simulink model "MCU_vectorControl_dsPIC33CK_LVMC"  (R2023a)
settings: Solver=FixedStepDiscrete  StartTime=0.0  StopTime=10.0  FixedStep=5e-5  RelTol=1e-3  EnableMultiTasking=on
undefined symbols (not defined in the file or in its folder): A0, A4, AN0, AN1, B0, B2, Bias1, Bias2, C12, C13, C14, C7, control, D11, D12, D13, D14, D5, D6, D7, diff, DiscIntNeverNeededParam, inverter, Max, MaxPer, model, ms, NumBits1, NumBits2, P20, P32, P55, P60, P61, P62, P69, P70, P71, P75, P76, P77, P78, Pin, pmsm, PosRange1, PosRange2, PWM1max, Resol, s, Slope1, Slope2, us
libraries: simulink x47, MCHP_Blockset x24
(part 3 of 4)

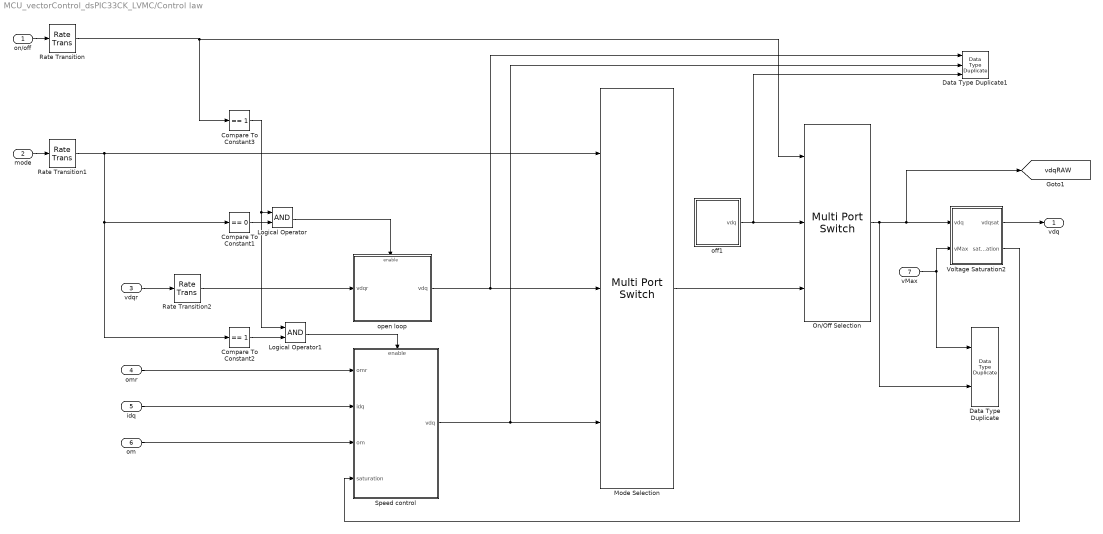
== system MCU_vectorControl_dsPIC33CK_LVMC/Control law ==
  on/off : Inport
  mode : Inport  Port=2
  vdqr : Inport  Port=3
  omr : Inport  Port=4
  idq : Inport  Port=5
  om : Inport  Port=6
  vMax : Inport  Port=7
  Compare To Constant1 : simulink/Logic and Bit Operations/Compare To Constant  relop===  const=0  OutDataTypeStr=boolean
  Compare To Constant2 : simulink/Logic and Bit Operations/Compare To Constant  relop===  const=1  OutDataTypeStr=boolean
  Compare To Constant3 : simulink/Logic and Bit Operations/Compare To Constant  relop===  const=1  OutDataTypeStr=boolean
  Data Type Duplicate : DataTypeDuplicate
  Data Type Duplicate1 : DataTypeDuplicate  NumInputPorts=3
  Logical Operator : Logic  AllPortsSameDT=off  OutDataTypeStr=boolean
  Logical Operator1 : Logic  AllPortsSameDT=off  OutDataTypeStr=boolean
  Mode Selection : MultiPortSwitch  DataPortOrder=Zero-based contiguous  Inputs=2  DiagnosticForDefault=None  zeroidx=on  SaturateOnIntegerOverflow=off  InputSameDT=off
  On/Off Selection : MultiPortSwitch  DataPortOrder=Zero-based contiguous  Inputs=2  DiagnosticForDefault=None  zeroidx=on  SaturateOnIntegerOverflow=off  InputSameDT=off
  Rate Transition : RateTransition
  Rate Transition1 : RateTransition
  Rate Transition2 : RateTransition
  Speed control : Subsystem
      settings: LibrarySourceBlock=insa_control_base/Current Control  PortSchema="{\"entries\":[{\"content\":{\"sides\":[{\"content\":{\"connectorIds\":[\"In1\",\"In2\",\"In3\",\"In4\"]},\"type\":\"ConnectorPlacement.EquallySpacedRectSide\",\"uuid\":\"e7aaa2d5-acdd-4a4d-91b1-423dc6f26e4f\"},{\"content\":{\"connectorIds\":[\"Out1\"],\"side\":\"RIGHT\"},\"type\":\"ConnectorPlacement.EquallySpacedRectSide\",\"uuid\":\"81691e4d-c138-404c-a913-2433211e99ad\"},{\"content\":{\"connectorIds\":[\"In5\"],\"side\":\"TOP\"},\"type\":\"ConnectorPlacement.EquallySpacedRectSide\",\"uuid\":\"67eaf657-96ad-4741-9677-f3dc17f9f096\"}]},\"type\":\"ConnectorPlacement.EquallySpacedConnector\",\"uuid\":\"09d68ba6-6bd5-4801-b033-56cd43b3cecf\"}],\"packageUris\":[\"http://schema.mathworks.com/mf0/Connector/R2020b\"],\"version\":\"1.0\"}"
  Voltage Saturation2 : Subsystem
  off1 : Subsystem
  open loop : Subsystem
  vdq : Outport  VectorParamsAs1DForOutWhenUnconnected=off
  tag scope: vdqRAW=global
  wires:
  Speed control/1(vdq) -> Data Type Duplicate1/2, Mode Selection/3
  Voltage Saturation2/2(saturation) -> Speed control/4(saturation)
  idq/1 -> Speed control/2(idq)
  om/1 -> Speed control/3(om)
  Logical Operator1/1 -> Speed control/5(enable)
  Compare To Constant3/1 -> Logical Operator/1, Logical Operator1/1
  Compare To Constant1/1 -> Logical Operator/2
  vdqr/1 -> Rate Transition2/1
  on/off/1 -> Rate Transition/1
  open loop/1(vdq) -> Mode Selection/2, Data Type Duplicate1/1
  off1/1(vdq) -> Data Type Duplicate1/3, On/Off Selection/2
  Mode Selection/1 -> On/Off Selection/3
  On/Off Selection/1 -> [vdqRAW], Voltage Saturation2/1(vdq), Data Type Duplicate/2
  vMax/1 -> Data Type Duplicate/1, Voltage Saturation2/2(vMax)
  Logical Operator/1 -> open loop/Enable
  Compare To Constant2/1 -> Logical Operator1/2
  mode/1 -> Rate Transition1/1
  Voltage Saturation2/1(vdqsat) -> vdq/1
  Rate Transition/1 -> Compare To Constant3/1, On/Off Selection/1
  Rate Transition1/1 -> Mode Selection/1, Compare To Constant2/1, Compare To Constant1/1
  Rate Transition2/1 -> open loop/1(vdqr)
  omr/1 -> Speed control/1(omr)

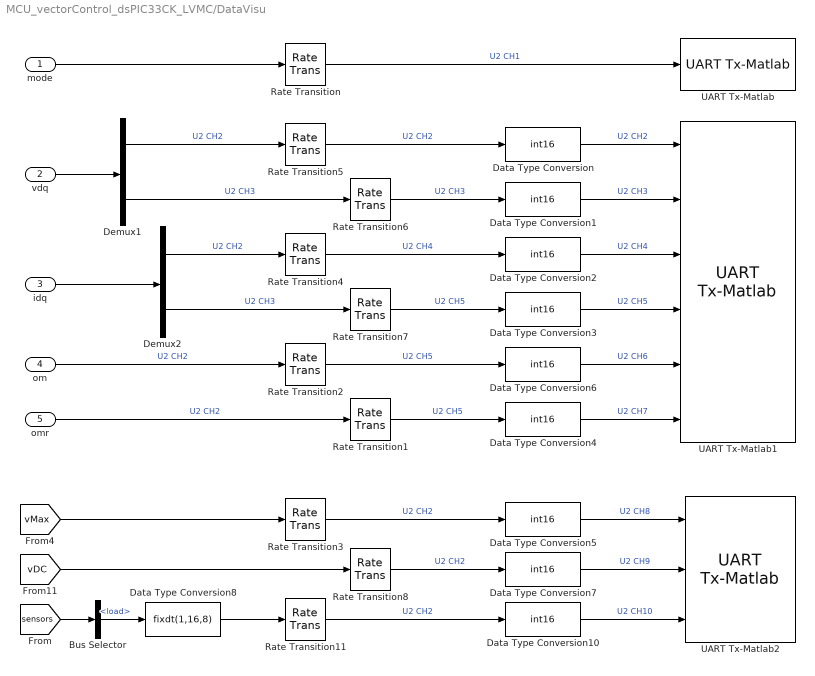
== system MCU_vectorControl_dsPIC33CK_LVMC/DataVisu ==
  mode : Inport
  vdq : Inport  Port=2
  idq : Inport  Port=3
  om : Inport  Port=4
  omr : Inport  Port=5
  Bus Selector : BusSelector  OutputSignals=MCU.load
  Data Type Conversion{,1..7,10} (9 alike) : DataTypeConversion  OutDataTypeStr=int16  ConvertRealWorld=Stored Integer (SI)  SaturateOnIntegerOverflow=off  RndMeth=Floor
  Data Type Conversion8 : DataTypeConversion  OutDataTypeStr=fixdt(1,16,8)  SaturateOnIntegerOverflow=off  RndMeth=Floor
  Demux1 : Demux  Outputs=2
  Demux2 : Demux  Outputs=2
  Rate Transition{,1..8,11} (10 alike) : RateTransition
  UART Tx-Matlab : MCHP_Blockset/BUS UART/UART Tx-Matlab  UART_REF=2  CHANNELS=[1]  AllOrNothing=off  SampleTime=.01  MCHP_MASTERLINK=MCU_vectorControl_dsPIC33CK_LVMC/BOARD dsPIC33CK LVMC/Microchip Master  MCHP_COMPILED_INFO="CompiledSampleTime= [0.010000000000000000208   0 ];CompiledInportDataTypes=[  5 ];CompiledInportDataWidth=[1];"
      settings: SourceProductName=MPLAB Device Blocks for Simulink
  UART Tx-Matlab1 : MCHP_Blockset/BUS UART/UART Tx-Matlab  UART_REF=2  CHANNELS=[2:7]  AllOrNothing=off  SampleTime=0.0005  MCHP_MASTERLINK=MCU_vectorControl_dsPIC33CK_LVMC/BOARD dsPIC33CK LVMC/Microchip Master  MCHP_COMPILED_INFO="CompiledSampleTime= [0.00050000000000000001041   0 ];CompiledInportDataTypes=[  4   4   4   4   4   4 ];CompiledInportDataWidth=[1  1  1  1  1  1];"
      settings: SourceProductName=MPLAB Device Blocks for Simulink
  UART Tx-Matlab2 : MCHP_Blockset/BUS UART/UART Tx-Matlab  UART_REF=2  CHANNELS=[8:10]  AllOrNothing=off  SampleTime=.01  MCHP_MASTERLINK=MCU_vectorControl_dsPIC33CK_LVMC/BOARD dsPIC33CK LVMC/Microchip Master  MCHP_COMPILED_INFO="CompiledSampleTime= [0.010000000000000000208   0 ];CompiledInportDataTypes=[  4   4   4 ];CompiledInportDataWidth=[1  1  1];"
      settings: SourceProductName=MPLAB Device Blocks for Simulink
  wires:
  Data Type Conversion8/1 -> Rate Transition11/1
  [sensors] -> Bus Selector/1
  Rate Transition11/1 -> Data Type Conversion10/1  "U2 CH2"
  Data Type Conversion10/1 -> UART Tx-Matlab2/3  "U2 CH10"
  Bus Selector/1 -> Data Type Conversion8/1  "<load>"
  Rate Transition8/1 -> Data Type Conversion7/1  "U2 CH2"
  Rate Transition3/1 -> Data Type Conversion5/1  "U2 CH2"
  Data Type Conversion7/1 -> UART Tx-Matlab2/2  "U2 CH9"
  Data Type Conversion5/1 -> UART Tx-Matlab2/1  "U2 CH8"
  [vMax] -> Rate Transition3/1
  [vDC] -> Rate Transition8/1
  Rate Transition1/1 -> Data Type Conversion4/1  "U2 CH5"
  Data Type Conversion4/1 -> UART Tx-Matlab1/6  "U2 CH7"
  omr/1 -> Rate Transition1/1  "U2 CH2"
  mode/1 -> Rate Transition/1
  Rate Transition/1 -> UART Tx-Matlab/1  "U2 CH1"
  om/1 -> Rate Transition2/1  "U2 CH2"
  Data Type Conversion6/1 -> UART Tx-Matlab1/5  "U2 CH6"
  Rate Transition2/1 -> Data Type Conversion6/1  "U2 CH5"
  Data Type Conversion3/1 -> UART Tx-Matlab1/4  "U2 CH5"
  Data Type Conversion2/1 -> UART Tx-Matlab1/3  "U2 CH4"
  Data Type Conversion1/1 -> UART Tx-Matlab1/2  "U2 CH3"
  Data Type Conversion/1 -> UART Tx-Matlab1/1  "U2 CH2"
  Rate Transition7/1 -> Data Type Conversion3/1  "U2 CH5"
  Demux1/1 -> Rate Transition5/1  "U2 CH2"
  Rate Transition4/1 -> Data Type Conversion2/1  "U2 CH4"
  Rate Transition6/1 -> Data Type Conversion1/1  "U2 CH3"
  Demux1/2 -> Rate Transition6/1  "U2 CH3"
  Rate Transition5/1 -> Data Type Conversion/1  "U2 CH2"
  Demux2/1 -> Rate Transition4/1  "U2 CH2"
  Demux2/2 -> Rate Transition7/1  "U2 CH3"
  idq/1 -> Demux2/1
  vdq/1 -> Demux1/1

== system MCU_vectorControl_dsPIC33CK_LVMC/Heart-beat 5Hz Blinking ==
  Delay : Delay  DelayLength=1  InitialCondition=0  SampleTime=.1
  Logical Operator : Logic  Operator=NOT  AllPortsSameDT=off  OutDataTypeStr=boolean
  Rate Transition2 : RateTransition  Deterministic=off  OutPortSampleTime=0.01
  LED1 : Outport  VectorParamsAs1DForOutWhenUnconnected=off
  wires:
  Rate Transition2/1 -> LED1/1
  Logical Operator/1 -> Rate Transition2/1, Delay/1
  Delay/1 -> Logical Operator/1

== system MCU_vectorControl_dsPIC33CK_LVMC/Init Enc ==
  rho_cont : Inport
  Constant1 : Constant  Value=[0.5 0.5 0.5]  OutDataTypeStr=Inherit: Inherit via back propagation
  Constant2 : Constant  Value=[.6 .5 .5]  OutDataTypeStr=Inherit: Inherit via back propagation
  Data Type Duplicate : DataTypeDuplicate
  Rate Transition1 : RateTransition
  Rate Transition2 : RateTransition
  Rate Transition3 : RateTransition
  Switch : Switch  Criteria=u2 > Threshold  SaturateOnIntegerOverflow=off  InputSameDT=off
  Switch1 : Switch  Criteria=u2 > Threshold  SaturateOnIntegerOverflow=off  InputSameDT=off
  Wait 1s : Subsystem
  reset encoder : Outport
  PWM [0 1] : Outport  Port=2
  wires:
  Rate Transition2/1 -> Switch/2
  Rate Transition1/1 -> reset encoder/1
  Switch1/1 -> PWM [0 1]/1
  Constant1/1 -> Switch1/3
  Constant2/1 -> Switch/3
  Wait 1s/2(init done) -> Rate Transition2/1
  Switch/1 -> Data Type Duplicate/2, Switch1/1
  rho_cont/1 -> Switch/1, Data Type Duplicate/1
  Wait 1s/1(init enc) -> Rate Transition1/1
  [onoff] -> Wait 1s/Enable, Rate Transition3/1
  Rate Transition3/1 -> Switch1/2

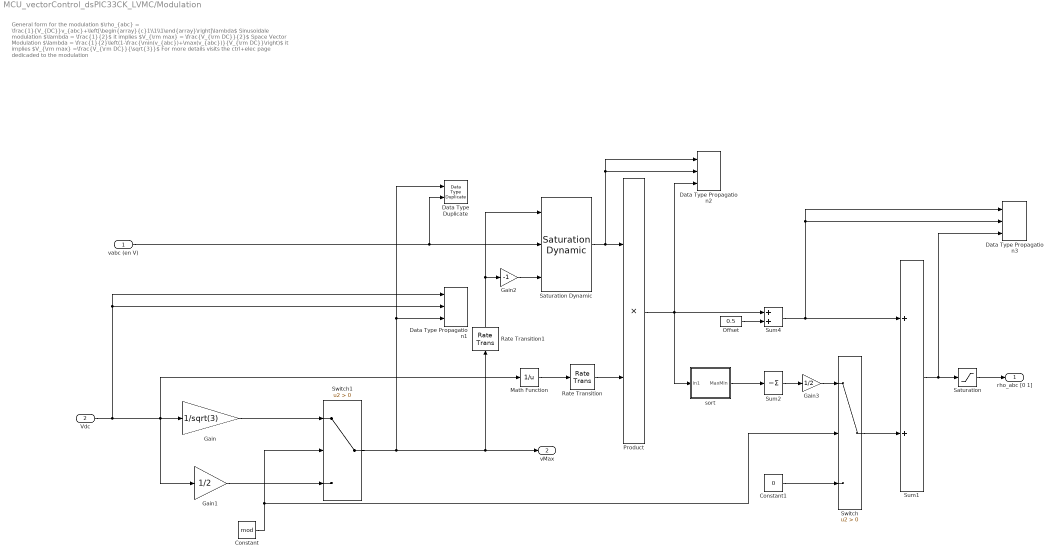
== system MCU_vectorControl_dsPIC33CK_LVMC/Modulation ==
  note: General form for the modulation
      | $\rho_{abc} = \frac{1}{V_{DC}}v_{abc}+\left[\begin{array}{c}1\\1\\1\end{array}\right]\lambda$
      | Sinusoidale modulation
      | $\lambda = \frac{1}{2}$ it implies $V_{\rm max} = \frac{V_{\rm DC}}{2}$
      | Space Vector Modulation
      | $\lambda = \frac{1}{2}\left(1-\frac{\min(v_{abc})+\max(v_{abc})}{V_{\rm DC}}\right)$ it implies $V_{\rm max} =\frac{V_{\rm DC}}{\sqrt{3}}$
      | For more details visits the ctrl+elec page dedicaded to the modulation
  "vabc (en V) " : Inport
  Vdc : Inport  Port=2
  Constant : Constant  Value=mod  OutDataTypeStr=boolean
  Constant1 : Constant  Value=0  OutDataTypeStr=Inherit: Inherit via back propagation
  Data Type Duplicate : DataTypeDuplicate
  Data Type Propagation1 : simulink/Signal Attributes/Data Type Propagation  PropDataType=fixdt(1, 16)  IfRefDouble=double  IfRefSingle=single  IsSigned=TRUE  NumBitsBase=max([NumBits1 NumBits2])  NumBitsMult=1  NumBitsAdd=0  NumBitsAllowFinal=[1:128]  PropScaling=2^-(15-ceil(log2(inverter.vDC/sqrt(3))))  ValuesUsedBestPrec=[100 -100]  SlopeBase=max([PosRange1 PosRange2])  SlopeMult=1/sqrt(3)  SlopeAdd=0  BiasBase=Bias1  BiasMult=1  BiasAdd=0
  Data Type Propagation2 : simulink/Signal Attributes/Data Type Propagation  PropDataType=fixdt(1, 16)  IfRefDouble=double  IfRefSingle=single  IsSigned=TRUE  NumBitsBase=max([NumBits1 NumBits2])  NumBitsMult=1  NumBitsAdd=0  NumBitsAllowFinal=[1:128]  PropScalingMode=Specify via dialog  PropScaling=2^-14  ValuesUsedBestPrec=[100 -100]  SlopeBase=Slope1/Slope2  SlopeMult=1  SlopeAdd=0  BiasBase=Bias1  BiasMult=1  BiasAdd=0
  Data Type Propagation3 : simulink/Signal Attributes/Data Type Propagation  PropDataType=fixdt(1, 16)  IfRefDouble=double  IfRefSingle=single  IsSigned=FALSE  NumBitsBase=max([NumBits1 NumBits2])  NumBitsMult=1  NumBitsAdd=0  NumBitsAllowFinal=[1:128]  PropScalingMode=Specify via dialog  PropScaling=2^-14  ValuesUsedBestPrec=[100 -100]  SlopeBase=Slope1/Slope2  SlopeMult=1  SlopeAdd=0  BiasBase=Bias1  BiasMult=1  BiasAdd=0
  Gain : Gain  Gain=1/sqrt(3)  OutDataTypeStr=Inherit: Same as input
  Gain1 : Gain  Gain=1/2  OutDataTypeStr=Inherit: Same as input
  Gain2 : Gain  Gain=-1  ParamDataTypeStr=int16  OutDataTypeStr=Inherit: Inherit via back propagation
  Gain3 : Gain  Gain=1/2  OutDataTypeStr=Inherit: Same as input
  Math Function : Math  Operator=reciprocal  OutputSignalType=real  OutDataTypeStr=fixdt(0,16,16)  SaturateOnIntegerOverflow=off
  "Offset " : Constant  Value=0.5  OutMin=[0]  OutMax=[1]  OutDataTypeStr=Inherit: Inherit via back propagation
  Product : Product  Inputs=**  OutDataTypeStr=Inherit: Inherit via back propagation  SaturateOnIntegerOverflow=on
  Rate Transition : RateTransition
  Rate Transition1 : RateTransition
  Saturation : Saturate  UpperLimit=1  LowerLimit=0
  Saturation Dynamic : simulink/Discontinuities/Saturation Dynamic  OutMin=[]  OutMax=[]  OutDataTypeStr=Inherit: Same as second input  OutDataType=fixdt(1, 16)  OutScaling=2^-10  DoSatur=off
  Sum1 : Sum  InputSameDT=on  OutMin=[0]  OutMax=[1]  OutDataTypeStr=Inherit: Inherit via back propagation  SaturateOnIntegerOverflow=on
  Sum2 : Sum  Inputs=-  InputSameDT=on  OutMin=[-1]  OutMax=[1]  SaturateOnIntegerOverflow=on  OutDataTypeStr=Inherit: Same as first input
  Sum4 : Sum  InputSameDT=on  OutMin=[-1]  OutMax=[1]  SaturateOnIntegerOverflow=on  OutDataTypeStr=Inherit: Same as first input
  Switch : Switch  Criteria=u2 > Threshold  SaturateOnIntegerOverflow=off  InputSameDT=off
  Switch1 : Switch  Criteria=u2 > Threshold  OutDataTypeStr=Inherit: Inherit via back propagation  SaturateOnIntegerOverflow=off  InputSameDT=off
  sort : Subsystem
  rho_abc [0 1] : Outport  VectorParamsAs1DForOutWhenUnconnected=off
  vMax : Outport  Port=2  VectorParamsAs1DForOutWhenUnconnected=off
  wires:
  Sum1/1 -> Saturation/1, Data Type Propagation3/3
  Vdc/1 -> Data Type Propagation1/2, Data Type Propagation1/1, Gain/1, Math Function/1, Gain1/1
  Gain3/1 -> Switch/1
  Saturation/1 -> rho_abc [0 1]/1
  Saturation Dynamic/1 -> Product/1, Data Type Propagation2/1, Data Type Propagation2/2
  Gain1/1 -> Switch1/3
  Gain/1 -> Switch1/1
  sort/1(MaxMin) -> Sum2/1
  Sum2/1 -> Gain3/1
  Sum4/1 -> Data Type Propagation3/2, Data Type Propagation3/1, Sum1/1
  Constant1/1 -> Switch/3
  Switch/1 -> Sum1/2
  "Offset "/1 -> Sum4/2
  Product/1 -> Data Type Propagation2/3, Sum4/1, sort/1(In1)
  Gain2/1 -> Saturation Dynamic/3
  Math Function/1 -> Rate Transition/1
  Switch1/1 -> Rate Transition1/1, vMax/1, Data Type Propagation1/3, Data Type Duplicate/1
  Constant/1 -> Switch1/2, Switch/2
  "vabc (en V) "/1 -> Data Type Duplicate/2, Saturation Dynamic/2
  Rate Transition/1 -> Product/2
  Rate Transition1/1 -> Saturation Dynamic/1, Gain2/1

== system MCU_vectorControl_dsPIC33CK_LVMC/Motor Choice + Gain Tunning ==

== system MCU_vectorControl_dsPIC33CK_LVMC/Park ==
  xab(c) : Inport
  P(pth) : Inport  Port=2
  Clarke : Subsystem
  Park : Subsystem
  idq : Outport
  wires:
  P(pth)/1 -> Park/2(P(pth))
  Park/1(xdq) -> idq/1  "idq"
  xab(c)/1 -> Clarke/1(xab(c))
  Clarke/1(xalphabeta) -> Park/1(xalphabeta)

== system MCU_vectorControl_dsPIC33CK_LVMC/Park inverse ==
  xdq : Inport
  P(pth) : Inport  Port=2
  Clarke Inverse : Subsystem
  Park inverse : Subsystem
  xabc : Outport
  wires:
  P(pth)/1 -> Park inverse/2(P(pth))
  Clarke Inverse/1(xabc) -> xabc/1
  xdq/1 -> Park inverse/1(xdq)
  Park inverse/1(xalpahbeta) -> Clarke Inverse/1(xalphabeta)

== system MCU_vectorControl_dsPIC33CK_LVMC/Rot ==
  sin cos : Inport
  Demux3 : Demux  Outputs=2
  Gain : Gain  Gain=-1  OutDataTypeStr=Inherit: Same as input
  Mux1 : Mux
  Reshape : Reshape  OutputDimensionality=Customize  OutputDimensions=[2,2]
  "cos sin -sin cos " : Outport  PortDimensions=[2 2]
  wires:
  Demux3/2 -> Mux1/1, Mux1/4
  Demux3/1 -> Gain/1, Mux1/3
  Mux1/1 -> Reshape/1
  Gain/1 -> Mux1/2
  sin cos/1 -> Demux3/1
  Reshape/1 -> "cos sin -sin cos "/1

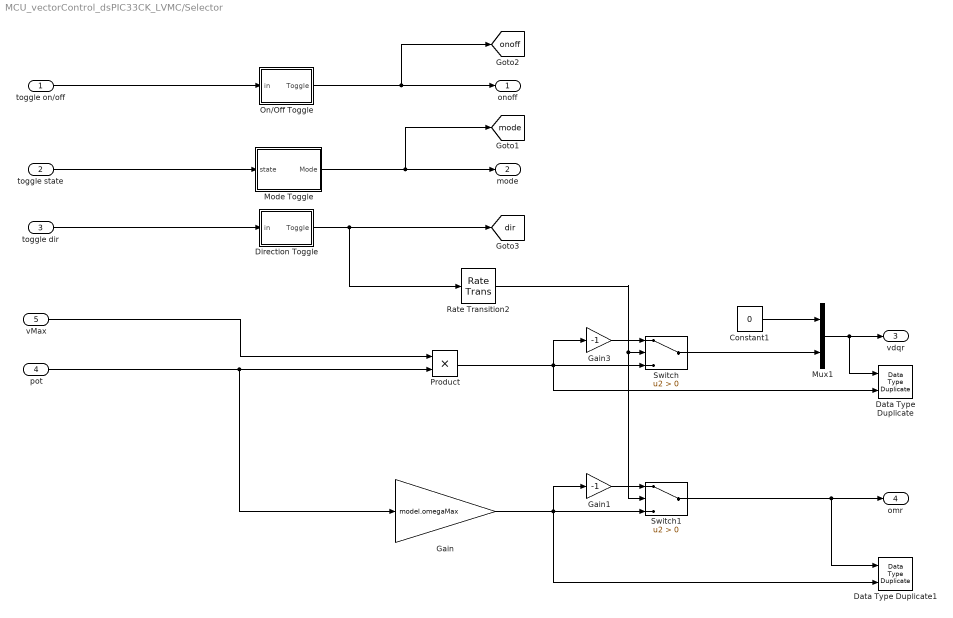
== system MCU_vectorControl_dsPIC33CK_LVMC/Selector ==
  toggle on/off : Inport  SampleTime=.01
  toggle state : Inport  Port=2  SampleTime=.01
  toggle dir : Inport  Port=3  SampleTime=.01
  pot : Inport  Port=4
  vMax : Inport  Port=5
  Constant1 : Constant  Value=0  OutDataTypeStr=Inherit: Inherit via back propagation
  Data Type Duplicate : DataTypeDuplicate
  Data Type Duplicate1 : DataTypeDuplicate
  Direction Toggle : Subsystem
  Gain : Gain  Gain=model.omegaMax  OutDataTypeStr=Inherit: Inherit via back propagation
  Gain1 : Gain  Gain=-1  OutDataTypeStr=Inherit: Inherit via back propagation  SaturateOnIntegerOverflow=on
  Gain3 : Gain  Gain=-1  OutDataTypeStr=Inherit: Inherit via back propagation  SaturateOnIntegerOverflow=on
  Mode Toggle : Subsystem
  Mux1 : Mux  Inputs=2
  On/Off Toggle : Subsystem
  Product : Product  OutDataTypeStr=Inherit: Same as first input
  Rate Transition2 : RateTransition  Integrity=off  OutPortSampleTime=0.001
  Switch : Switch  Criteria=u2 > Threshold  OutDataTypeStr=Inherit: Inherit via back propagation  SaturateOnIntegerOverflow=off  InputSameDT=off
  Switch1 : Switch  Criteria=u2 > Threshold  OutDataTypeStr=Inherit: Inherit via back propagation  SaturateOnIntegerOverflow=off  InputSameDT=off
  onoff : Outport
  mode : Outport  Port=2
  vdqr : Outport  Port=3  VectorParamsAs1DForOutWhenUnconnected=off
  omr : Outport  Port=4  VectorParamsAs1DForOutWhenUnconnected=off
  tag scope: dir=global, mode=global, onoff=global
  wires:
  Switch1/1 -> omr/1, Data Type Duplicate1/1
  Direction Toggle/1(Toggle) -> Rate Transition2/1, [dir]
  Gain1/1 -> Switch1/1
  Gain/1 -> Gain1/1, Switch1/3, Data Type Duplicate1/2
  Product/1 -> Data Type Duplicate/2, Switch/3, Gain3/1
  Mux1/1 -> Data Type Duplicate/1, vdqr/1
  Constant1/1 -> Mux1/1
  toggle on/off/1 -> On/Off Toggle/1(in)
  On/Off Toggle/1(Toggle) -> [onoff], onoff/1
  Mode Toggle/1(Mode) -> [mode], mode/1
  toggle state/1 -> Mode Toggle/1(state)
  toggle dir/1 -> Direction Toggle/1(in)
  Gain3/1 -> Switch/1
  Switch/1 -> Mux1/2
  vMax/1 -> Product/1
  Rate Transition2/1 -> Switch/2, Switch1/2
  pot/1 -> Gain/1, Product/2

== system MCU_vectorControl_dsPIC33CK_LVMC/BOARD dsPIC33CK LVMC/ADC ==
  ADC dsPIC High Speed SAR Motor Currents : MCHP_Blockset/Analog IO/ADC dsPIC High Speed SAR  ACLKCON=Optimized for PWM resolution & ADC conversion speed  ADC_FRACT=Fractional (left aligned)  ADC_NRE=off  DMA_Size=Single trigger - (default)  ADC_Synchronisation=Triggered by custom source  ADC_Trig=Dynamic Options  ADC_Trig_TXT=PWM1 Trigger 1  ADC_TrigTimeStep=Trig model step after all sample from this block are converted  ADC_TrigInfo=0  SampleTime=50e-6  S_INPUT=[]  S_INPUT_Size=[]  S_OUTPUT="[5  5]"  S_OUTPUT_Size="[1  1]"  S_ListCustomDatatype=S.S_ListCustomDatatype={};  MCHP_USER_INTERRUPTS={ADCAN0}{ADCBUF0}{ADC Data 0 Ready}{VectorName(ADCAN0Interrupt) Priority(-1) RegisterReadClear(ADCBUF0)Config_BitSet(ADIELbits.IE0) };{ADCAN1}{ADCBUF1}{ADC Data 1 Ready}{VectorName(ADCAN1Interrupt) Priority(-1) RegisterReadClear(ADCBUF1)Config_BitSet(ADIELbits.IE1) };  MCHP_PORT={Analog Input 0}{AN0}15:2:A0;{Analog Input 1}{AN1}15:2:B2;  MCHP_MASTERLINK=MCU_vectorControl_dsPIC33CK_LVMC/BOARD dsPIC33CK LVMC/Microchip Master  MCHP_CRC=3824902  ADC_Info=Total Time = 640(ns)  ADC0_pin=Dynamic Options  ADC0_pin_TXT=AN0 / A0 / Pin[16]  ADC0_R="< 5    kOhm"  ADC0_res=12 bits  ADC0_signed=signed 16 bits  ADC0_FILTER=No Oversampling  ADC0_FILTER_nSamples=256 samples  ADC0_STRGEN=Start sampling followed by conversion  ADC0_STRGEN_on=Start sampling followed by conversion  ADC0_SSAMPEN=off  ADC0_Info=tSmp_min=260(ns) x 1 = 260(ns) ; tConv=370(ns) x 1 = 370(ns) ; TOTAL=640(ns)  ADC1_pin=Dynamic Options  ADC1_pin_TXT=AN1 / B2 / Pin[41]  ADC1_R="< 5    kOhm"  ADC1_res=12 bits  ADC1_signed=signed 16 bits  ADC1_FILTER=No Oversampling  ADC1_FILTER_nSamples=128 samples  ADC1_STRGEN=Start sampling followed by conversion  ADC1_STRGEN_on=Start sampling followed by conversion  ADC1_SSAMPEN=off  ADC1_Info=tSmp_min=260(ns) x 1 = 260(ns) ; tConv=370(ns) x 1 = 370(ns) ; TOTAL=640(ns)  ADC2_pin=Dynamic Options  ADC2_pin_TXT=Not used  ADC2_R="< 5    kOhm"  ADC2_res=12 bits  ADC2_signed=signed 16 bits  ADC2_FILTER=No Oversampling  ADC2_FILTER_nSamples=256 samples  ADC2_STRGEN=End sampling and start conversion  ADC2_STRGEN_on=Start sampling followed by conversion  ADC2_SSAMPEN=on  ADC2_Info=tSmp_min=14.706(ns) x 0 = 0(s) ; tConv=154.41(ns) x 0 = 0(s) ; TOTAL=0(s)  ADC3_pin=Dynamic Options  ADC3_pin_TXT=Not used  ADC3_R="< 10   kOhm"  ADC3_res=12 bits  ADC3_signed=signed 16 bits  ADC3_FILTER=Burst convert of n samples are Summed  ADC3_FILTER_nSamples=64 samples  ADC3_STRGEN=End sampling and start conversion  ADC3_STRGEN_on=Start sampling followed by conversion  ADC3_SSAMPEN=on  ADC3_Info=tSmp_min=14.706(ns) x 0 = 0(s) ; tConv=154.41(ns) x 0 = 0(s) ; TOTAL=0(s)  ADC4_pin=Dynamic Options  ADC4_pin_TXT=Not used  ADC4_R=< 200 Ohm  ADC4_res=12 bits  ADC4_signed=unsigned 16 bits  ADC4_FILTER=No Oversampling  ADC4_FILTER_nSamples=256 samples  ADC4_STRGEN=End sampling and start conversion  ADC4_STRGEN_on=Start sampling followed by conversion  ADC4_SSAMPEN=off  ADC4_Info=tSmp_min=14.706(ns) x 0 = 0(s) ; tConv=154.41(ns) x 0 = 0(s) ; TOTAL=0(s)  ADC5_pin=Dynamic Options  ADC5_pin_TXT=Not used  ADC5_R=< 200 Ohm  ADC5_res=12 bits  ADC5_signed=unsigned 16 bits  ADC5_FILTER=Burst convert of n samples are Summed  ADC5_FILTER_nSamples=256 samples  ADC5_STRGEN=End sampling and start conversion  ADC5_STRGEN_on=Start sampling followed by conversion  ADC5_SSAMPEN=on  ADC5_Info=tSmp_min=14.706(ns) x 0 = 0(s) ; tConv=154.41(ns) x 0 = 0(s) ; TOTAL=0(s)  ADC6_pin=Dynamic Options  ADC6_pin_TXT=Not used  ADC6_R=< 200 Ohm  ADC6_res=12 bits  ADC6_signed=unsigned 16 bits  ADC6_FILTER=Burst convert of n samples are Summed  ADC6_FILTER_nSamples=256 samples  ADC6_STRGEN=End sampling and start conversion  ADC6_STRGEN_on=Start sampling followed by conversion  ADC6_SSAMPEN=on  ADC6_Info=tSmp_min=14.706(ns) x 0 = 0(s) ; tConv=154.41(ns) x 0 = 0(s) ; TOTAL=0(s)  ADC7_R="< 5    kOhm"  ADC7_res=12 bits  ADC7_AN0=Not used  ADC7_AN1=Not used  ADC7_AN2=Not used  ADC7_AN3=Not used  ADC7_AN4=Not used  ADC7_AN5=Not used  ADC7_AN6=Not used  ADC7_AN7=Not used  ADC7_AN8=Not used  ADC7_AN9=Not used  ADC7_AN10=Not used  ADC7_AN11=Not used  ADC7_AN12=Not used  ADC7_AN13=Not used  ADC7_AN14=Not used  ADC7_AN15=Not used  ADC7_AN16=Not used  ADC7_AN17=Not used  ADC7_AN18=Not used  ADC7_AN19=Not used  ADC7_AN20=Not used  ADC7_AN21=Not used  ADC7_AN22=Not used  ADC7_AN23=Not used  ADC7_AN24=Not used  ADC7_AN25=Not used  ADC7_AN26=Not used  ADC7_AN27=Not used  ADC7_AN28=Not used  ADC7_AN29=Not used  ADC7_AN30=Not used  ADC7_AN31=Not used  IVref=Not used  IVTemp=Not used  ADC7_Info=tSmp_min=20(ns) x 0 = 0(s) ; tConv=210(ns) x 0 = 0(s) ; TOTAL=0(s)
      settings: SourceProductName=MPLAB Device Blocks for Simulink
  ADC dsPIC High Speed SAR others : MCHP_Blockset/Analog IO/ADC dsPIC High Speed SAR  ACLKCON=Not used  ADC_FRACT=Fractional (left aligned)  ADC_NRE=off  DMA_Size=Single trigger - (default)  ADC_Synchronisation=Triggered by custom source  ADC_Trig=Dynamic Options  ADC_Trig_TXT=PWM1 Trigger 1  ADC_TrigTimeStep=None (independant)  ADC_TrigInfo=0  SampleTime=50e-6  S_INPUT=[]  S_INPUT_Size=[]  S_OUTPUT="[5  5]"  S_OUTPUT_Size="[1  1]"  S_ListCustomDatatype=S.S_ListCustomDatatype={};  MCHP_USER_INTERRUPTS={ADCAN3}{ADCBUF3}{ADC Data 3 Ready}{VectorName(ADCAN3Interrupt) Priority(-1) RegisterReadClear(ADCBUF3)Config_BitSet(ADIELbits.IE3) };{ADCAN10}{ADCBUF10}{ADC Data 10 Ready}{VectorName(ADCAN10Interrupt) Priority(-1) RegisterReadClear(ADCBUF10)Config_BitSet(ADIELbits.IE10) };{ADCAN14}{ADCBUF14}{ADC Data 14 Ready}{VectorName(ADCAN14Interrupt) Priority(-1) RegisterReadClear(ADCBUF14)Config_BitSet(ADIELbits.IE14) };  MCHP_PORT={Analog Input 4}{AN4}15:2:A4;{Analog Input 11}{AN11}15:2:B9;{Analog Input 15}{AN15}15:2:C3;  MCHP_MASTERLINK=MCU_vectorControl_dsPIC33CK_LVMC/BOARD dsPIC33CK LVMC/Microchip Master  MCHP_CRC=3970270  ADC_Info=Total Time = 1.98(us)  ADC0_pin=Dynamic Options  ADC0_pin_TXT=Not used  ADC0_R="< 5    kOhm"  ADC0_res=12 bits  ADC0_signed=signed 16 bits  ADC0_FILTER=No Oversampling  ADC0_FILTER_nSamples=256 samples  ADC0_STRGEN=Start sampling followed by conversion  ADC0_STRGEN_on=Start sampling followed by conversion  ADC0_SSAMPEN=off  ADC0_Info=tSmp_min=20(ns) x 0 = 0(s) ; tConv=210(ns) x 0 = 0(s) ; TOTAL=0(s)  ADC1_pin=Dynamic Options  ADC1_pin_TXT=Not used  ADC1_R="< 5    kOhm"  ADC1_res=12 bits  ADC1_signed=signed 16 bits  ADC1_FILTER=No Oversampling  ADC1_FILTER_nSamples=128 samples  ADC1_STRGEN=Start sampling followed by conversion  ADC1_STRGEN_on=Start sampling followed by conversion  ADC1_SSAMPEN=off  ADC1_Info=tSmp_min=20(ns) x 0 = 0(s) ; tConv=210(ns) x 0 = 0(s) ; TOTAL=0(s)  ADC2_pin=Dynamic Options  ADC2_pin_TXT=Not used  ADC2_R="< 5    kOhm"  ADC2_res=12 bits  ADC2_signed=signed 16 bits  ADC2_FILTER=No Oversampling  ADC2_FILTER_nSamples=256 samples  ADC2_STRGEN=End sampling and start conversion  ADC2_STRGEN_on=Start sampling followed by conversion  ADC2_SSAMPEN=on  ADC2_Info=tSmp_min=14.706(ns) x 0 = 0(s) ; tConv=154.41(ns) x 0 = 0(s) ; TOTAL=0(s)  ADC3_pin=Dynamic Options  ADC3_pin_TXT=Not used  ADC3_R="< 10   kOhm"  ADC3_res=12 bits  ADC3_signed=signed 16 bits  ADC3_FILTER=Burst convert of n samples are Summed  ADC3_FILTER_nSamples=64 samples  ADC3_STRGEN=End sampling and start conversion  ADC3_STRGEN_on=Start sampling followed by conversion  ADC3_SSAMPEN=on  ADC3_Info=tSmp_min=14.706(ns) x 0 = 0(s) ; tConv=154.41(ns) x 0 = 0(s) ; TOTAL=0(s)  ADC4_pin=Dynamic Options  ADC4_pin_TXT=Not used  ADC4_R=< 200 Ohm  ADC4_res=12 bits  ADC4_signed=unsigned 16 bits  ADC4_FILTER=No Oversampling  ADC4_FILTER_nSamples=256 samples  ADC4_STRGEN=End sampling and start conversion  ADC4_STRGEN_on=Start sampling followed by conversion  ADC4_SSAMPEN=off  ADC4_Info=tSmp_min=14.706(ns) x 0 = 0(s) ; tConv=154.41(ns) x 0 = 0(s) ; TOTAL=0(s)  ADC5_pin=Dynamic Options  ADC5_pin_TXT=Not used  ADC5_R=< 200 Ohm  ADC5_res=12 bits  ADC5_signed=unsigned 16 bits  ADC5_FILTER=Burst convert of n samples are Summed  ADC5_FILTER_nSamples=256 samples  ADC5_STRGEN=End sampling and start conversion  ADC5_STRGEN_on=Start sampling followed by conversion  ADC5_SSAMPEN=on  ADC5_Info=tSmp_min=14.706(ns) x 0 = 0(s) ; tConv=154.41(ns) x 0 = 0(s) ; TOTAL=0(s)  ADC6_pin=Dynamic Options  ADC6_pin_TXT=Not used  ADC6_R=< 200 Ohm  ADC6_res=12 bits  ADC6_signed=unsigned 16 bits  ADC6_FILTER=Burst convert of n samples are Summed  ADC6_FILTER_nSamples=256 samples  ADC6_STRGEN=End sampling and start conversion  ADC6_STRGEN_on=Start sampling followed by conversion  ADC6_SSAMPEN=on  ADC6_Info=tSmp_min=14.706(ns) x 0 = 0(s) ; tConv=154.41(ns) x 0 = 0(s) ; TOTAL=0(s)  ADC7_R="< 5    kOhm"  ADC7_res=12 bits  ADC7_AN0=Not used  ADC7_AN1=Not used  ADC7_AN2=Not used  ADC7_AN3=Not used  ADC7_AN4=signed int16  ADC7_AN5=Not used  ADC7_AN6=Not used  ADC7_AN7=Not used  ADC7_AN8=Not used  ADC7_AN9=Not used  ADC7_AN10=Not used  ADC7_AN11=unsigned int16  ADC7_AN12=Not used  ADC7_AN13=Not used  ADC7_AN14=Not used  ADC7_AN15=unsigned int16  ADC7_AN16=Not used  ADC7_AN17=Not used  ADC7_AN18=Not used  ADC7_AN19=Not used  ADC7_AN20=Not used  ADC7_AN21=Not used  ADC7_AN22=Not used  ADC7_AN23=Not used  ADC7_AN24=Not used  ADC7_AN25=Not used  ADC7_AN26=Not used  ADC7_AN27=Not used  ADC7_AN28=Not used  ADC7_AN29=Not used  ADC7_AN30=Not used  ADC7_AN31=Not used  IVref=Not used  IVTemp=Not used  ADC7_Info=tSmp_min=280(ns) x 3 = 840(ns) ; tConv=370(ns) x 3 = 1.11(us) ; TOTAL=1.98(us)
      settings: SourceProductName=MPLAB Device Blocks for Simulink
  Ia : Outport  VectorParamsAs1DForOutWhenUnconnected=off
  Ib : Outport  Port=2  VectorParamsAs1DForOutWhenUnconnected=off
  IBus : Outport  Port=3  VectorParamsAs1DForOutWhenUnconnected=off
  pot : Outport  Port=4  VectorParamsAs1DForOutWhenUnconnected=off
  V_BUS : Outport  Port=5  VectorParamsAs1DForOutWhenUnconnected=off
  wires:
  ADC dsPIC High Speed SAR Motor Currents/2 -> Ib/1
  ADC dsPIC High Speed SAR Motor Currents/1 -> Ia/1
  ADC dsPIC High Speed SAR others/1 -> IBus/1
  ADC dsPIC High Speed SAR others/2 -> pot/1
  ADC dsPIC High Speed SAR others/3 -> V_BUS/1

== system MCU_vectorControl_dsPIC33CK_LVMC/BOARD dsPIC33CK LVMC/Center & sign reversal ==
  I_ab : Inport
  Bias Update : Inport  Port=2
  Average and Sign reverse : Sum  Inputs=+-  OutDataTypeStr=Inherit: Same as accumulator  SaturateOnIntegerOverflow=on
  Downsample Averaged 2000 samples remove bias : Subsystem  mask{DownSample=2000}
      mask prompts: DownSample "DownSample Factor"
  Rate Transition1 : RateTransition  Integrity=off  Deterministic=off
  Iab : Outport
  wires:
  I_ab/1 -> Average and Sign reverse/2, Downsample Averaged 2000 samples remove bias/1(In1)
  Bias Update/1 -> Downsample Averaged 2000 samples remove bias/Enable
  Downsample Averaged 2000 samples remove bias/1(Out1) -> Rate Transition1/1
  Rate Transition1/1 -> Average and Sign reverse/1
  Average and Sign reverse/1 -> Iab/1  "I_ab_raw"

== system MCU_vectorControl_dsPIC33CK_LVMC/BOARD dsPIC33CK LVMC/Downsample Averaged x20 ==
  note: DownSample & Average by changing data scaling
  In1 : Inport
  Compare To Constant : simulink/Logic and Bit Operations/Compare To Constant  relop===  const=1  OutDataTypeStr=boolean
  Counter Limited : simulink/Sources/Counter Limited  uplimit=DownSample-1  tsamp=-1
  Data Type Duplicate : DataTypeDuplicate
  Data Type Propagation : simulink/Signal Attributes/Data Type Propagation  PropDataType=fixdt(1, 16)  IfRefDouble=double  IfRefSingle=single  IsSigned=IsSigned1 or IsSigned2  NumBitsBase=NumBits1+NumBits2  NumBitsMult=1  NumBitsAdd=0  NumBitsAllowFinal=1:128  PropScaling=2^-10  ValuesUsedBestPrec=[5 -7]  SlopeBase=Slope1  SlopeMult=1  SlopeAdd=0  BiasBase=Bias1  BiasMult=1  BiasAdd=0
  Data Type Propagation1 : simulink/Signal Attributes/Data Type Propagation  PropDataType=fixdt(1, 16)  IfRefDouble=double  IfRefSingle=single  IsSigned=IsSigned1 or IsSigned2  NumBitsBase=NumBits1+NumBits2  NumBitsMult=1  NumBitsAdd=0  NumBitsAllowFinal=1:128  PropScaling=2^-10  ValuesUsedBestPrec=[5 -7]  SlopeBase=PosRange1  SlopeMult=1  SlopeAdd=0  BiasBase=Bias1  BiasMult=1  BiasAdd=0
  Discrete-Time Integrator : DiscreteIntegrator  IntegratorMethod=Accumulation: Backward Euler  gainval=1  ExternalReset=sampled level  SampleTime=-1  OutDataTypeStr=Inherit: Inherit via back propagation  ICPrevOutput=DiscIntNeverNeededParam  ICPrevScaledInput=DiscIntNeverNeededParam
  Gain : Gain  Gain=1/DownSample  OutDataTypeStr=Inherit: Inherit via back propagation  RndMeth=Round
  Gain1 : Gain  Gain=1/DownSample  OutDataTypeStr=Inherit: Inherit via back propagation
  Rate Transition1 : RateTransition  OutPortSampleTimeOpt=Multiple of input port sample time  OutPortSampleTimeMultiple=DownSample  OutPortSampleTime=DownSample
  Rate Transition3 : RateTransition  OutPortSampleTimeOpt=Multiple of input port sample time  OutPortSampleTimeMultiple=DownSample  OutPortSampleTime=DownSample
  Terminator : Terminator
  Out1 : Outport  VectorParamsAs1DForOutWhenUnconnected=off
  wires:
  Gain1/1 -> Data Type Propagation1/3, Terminator/1
  Rate Transition1/1 -> Data Type Duplicate/1, Data Type Propagation1/1, Data Type Propagation1/2
  Gain/1 -> Out1/1, Data Type Duplicate/2
  Counter Limited/1 -> Compare To Constant/1
  Discrete-Time Integrator/1 -> Rate Transition3/1, Data Type Propagation/3
  Compare To Constant/1 -> Discrete-Time Integrator/2
  In1/1 -> Data Type Propagation/1, Data Type Propagation/2, Discrete-Time Integrator/1, Rate Transition1/1
  Rate Transition3/1 -> Gain/1, Gain1/1

== system MCU_vectorControl_dsPIC33CK_LVMC/BOARD dsPIC33CK LVMC/Downsample x20 ==
  note: DownSample & Average by changing data scaling
  In1 : Inport
  Compare To Constant : simulink/Logic and Bit Operations/Compare To Constant  relop===  const=1  OutDataTypeStr=boolean
  Counter Limited : simulink/Sources/Counter Limited  uplimit=DownSample-1  tsamp=-1
  Data Type Duplicate : DataTypeDuplicate
  Data Type Propagation : simulink/Signal Attributes/Data Type Propagation  PropDataType=fixdt(1, 16)  IfRefDouble=double  IfRefSingle=single  IsSigned=IsSigned1 or IsSigned2  NumBitsBase=NumBits1+NumBits2  NumBitsMult=1  NumBitsAdd=0  NumBitsAllowFinal=1:128  PropScaling=2^-10  ValuesUsedBestPrec=[5 -7]  SlopeBase=Slope1  SlopeMult=1  SlopeAdd=0  BiasBase=Bias1  BiasMult=1  BiasAdd=0
  Data Type Propagation1 : simulink/Signal Attributes/Data Type Propagation  PropDataType=fixdt(1, 16)  IfRefDouble=double  IfRefSingle=single  IsSigned=IsSigned1 or IsSigned2  NumBitsBase=NumBits1+NumBits2  NumBitsMult=1  NumBitsAdd=0  NumBitsAllowFinal=1:128  PropScaling=2^-10  ValuesUsedBestPrec=[5 -7]  SlopeBase=PosRange1  SlopeMult=1  SlopeAdd=0  BiasBase=Bias1  BiasMult=1  BiasAdd=0
  Discrete-Time Integrator : DiscreteIntegrator  IntegratorMethod=Accumulation: Backward Euler  gainval=1  ExternalReset=sampled level  SampleTime=-1  OutDataTypeStr=Inherit: Inherit via back propagation  ICPrevOutput=DiscIntNeverNeededParam  ICPrevScaledInput=DiscIntNeverNeededParam
  Gain : Gain  Gain=1/DownSample  OutDataTypeStr=Inherit: Inherit via back propagation  RndMeth=Round
  Gain1 : Gain  Gain=1/DownSample  OutDataTypeStr=Inherit: Inherit via back propagation
  Rate Transition1 : RateTransition  OutPortSampleTimeOpt=Multiple of input port sample time  OutPortSampleTimeMultiple=DownSample  OutPortSampleTime=DownSample
  Rate Transition3 : RateTransition  OutPortSampleTimeOpt=Multiple of input port sample time  OutPortSampleTimeMultiple=DownSample  OutPortSampleTime=DownSample
  Terminator : Terminator
  Out1 : Outport  VectorParamsAs1DForOutWhenUnconnected=off
  wires:
  Rate Transition3/1 -> Gain1/1, Gain/1
  In1/1 -> Rate Transition1/1, Discrete-Time Integrator/1, Data Type Propagation/2, Data Type Propagation/1
  Compare To Constant/1 -> Discrete-Time Integrator/2
  Discrete-Time Integrator/1 -> Data Type Propagation/3, Rate Transition3/1
  Counter Limited/1 -> Compare To Constant/1
  Gain/1 -> Data Type Duplicate/2, Out1/1
  Rate Transition1/1 -> Data Type Propagation1/2, Data Type Propagation1/1, Data Type Duplicate/1
  Gain1/1 -> Terminator/1, Data Type Propagation1/3

== system MCU_vectorControl_dsPIC33CK_LVMC/BOARD dsPIC33CK LVMC/Downsample x20 _ ==
  note: DownSample & Average by changing data scaling
  In1 : Inport
  Compare To Constant : simulink/Logic and Bit Operations/Compare To Constant  relop===  const=1  OutDataTypeStr=boolean
  Counter Limited : simulink/Sources/Counter Limited  uplimit=DownSample-1  tsamp=-1
  Data Type Duplicate : DataTypeDuplicate
  Data Type Propagation : simulink/Signal Attributes/Data Type Propagation  PropDataType=fixdt(1, 16)  IfRefDouble=double  IfRefSingle=single  IsSigned=IsSigned1 or IsSigned2  NumBitsBase=NumBits1+NumBits2  NumBitsMult=1  NumBitsAdd=0  NumBitsAllowFinal=1:128  PropScaling=2^-10  ValuesUsedBestPrec=[5 -7]  SlopeBase=Slope1  SlopeMult=1  SlopeAdd=0  BiasBase=Bias1  BiasMult=1  BiasAdd=0
  Data Type Propagation1 : simulink/Signal Attributes/Data Type Propagation  PropDataType=fixdt(1, 16)  IfRefDouble=double  IfRefSingle=single  IsSigned=IsSigned1 or IsSigned2  NumBitsBase=NumBits1+NumBits2  NumBitsMult=1  NumBitsAdd=0  NumBitsAllowFinal=1:128  PropScaling=2^-10  ValuesUsedBestPrec=[5 -7]  SlopeBase=PosRange1  SlopeMult=1  SlopeAdd=0  BiasBase=Bias1  BiasMult=1  BiasAdd=0
  Discrete-Time Integrator : DiscreteIntegrator  IntegratorMethod=Accumulation: Backward Euler  gainval=1  ExternalReset=sampled level  SampleTime=-1  OutDataTypeStr=Inherit: Inherit via back propagation  ICPrevOutput=DiscIntNeverNeededParam  ICPrevScaledInput=DiscIntNeverNeededParam
  Gain : Gain  Gain=1/DownSample  OutDataTypeStr=Inherit: Inherit via back propagation  RndMeth=Round
  Gain1 : Gain  Gain=1/DownSample  OutDataTypeStr=Inherit: Inherit via back propagation
  Rate Transition1 : RateTransition  OutPortSampleTimeOpt=Multiple of input port sample time  OutPortSampleTimeMultiple=DownSample  OutPortSampleTime=DownSample
  Rate Transition3 : RateTransition  OutPortSampleTimeOpt=Multiple of input port sample time  OutPortSampleTimeMultiple=DownSample  OutPortSampleTime=DownSample
  Terminator : Terminator
  Out1 : Outport  VectorParamsAs1DForOutWhenUnconnected=off
  wires:
  Gain1/1 -> Data Type Propagation1/3, Terminator/1
  Rate Transition1/1 -> Data Type Duplicate/1, Data Type Propagation1/1, Data Type Propagation1/2
  Gain/1 -> Out1/1, Data Type Duplicate/2
  Counter Limited/1 -> Compare To Constant/1
  Discrete-Time Integrator/1 -> Rate Transition3/1, Data Type Propagation/3
  Compare To Constant/1 -> Discrete-Time Integrator/2
  In1/1 -> Data Type Propagation/1, Data Type Propagation/2, Discrete-Time Integrator/1, Rate Transition1/1
  Rate Transition3/1 -> Gain/1, Gain1/1

== system MCU_vectorControl_dsPIC33CK_LVMC/BOARD dsPIC33CK LVMC/LVMC board webpage ==

== system MCU_vectorControl_dsPIC33CK_LVMC/BOARD dsPIC33CK LVMC/PWM Scaling ==
  vabc [0 1] : Inport
  Gain : Gain  Gain=PWM1max  OutDataTypeStr=uint16
  PWM : Outport  VectorParamsAs1DForOutWhenUnconnected=off
  wires:
  vabc [0 1]/1 -> Gain/1
  Gain/1 -> PWM/1

== system MCU_vectorControl_dsPIC33CK_LVMC/BOARD dsPIC33CK LVMC/Timing Analysis ==
  note: CPU overload is 0 if no overload took place between two MCU Overload block execution.
      | Otherwise, bits field output code for TID(s) responsible for at least one overload.
  Downsample Averaged2 : Subsystem  mask{InputSampleTime=.0005, DownSample=200}
      mask prompts: InputSampleTime "Input sample time"; DownSample "DownSample Factor"
  Gain : Gain  Gain=10e-9/.0005 * 100  OutMin=0  OutMax=100  OutDataTypeStr=fixdt(0,16)  RndMeth=Simplest  SaturateOnIntegerOverflow=on
  MCU Load : MCHP_Blockset/Profiling/MCU Load  MCULoadPin=Dynamic Options  MCULoadPin_TXT=None  MCULoadMeasure=on  TIMER_Resolution=Dynamic Options  TIMER_Resolution_TXT="Resol: 0.01(us)  -  Max: 0.655(ms)"  MCHP_TIMER_REQUEST={MCU_Load}{MCU_Load}21:5:0:0:[]:65536;  MCHP_TIMER_RESULT=[1 65535 ]  MCHP_MASTERLINK=MCU_vectorControl_dsPIC33CK_LVMC/BOARD dsPIC33CK LVMC/Microchip Master  MCHP_COMPILED_INFO="CompiledSampleTime= [0.00050000000000000001041   0 ];CompiledInportDataTypes=[    ];CompiledInportDataWidth=[];"  Info="Timer 1:  Resol: 10(ns)  -  Max: 655.36(us)"  SampleTime=.0005
      settings: SourceProductName=MPLAB Device Blocks for Simulink
  MCU Overload : MCHP_Blockset/Profiling/MCU Overload  MCUOverloadBlockOutput=on  MCUOverLoadPin=Dynamic Options  MCUOverLoadPin_TXT=None  MCHP_MASTERLINK=MCU_vectorControl_dsPIC33CK_LVMC/BOARD dsPIC33CK LVMC/Microchip Master  SampleTime=-1
      settings: SourceProductName=MPLAB Device Blocks for Simulink
  Overload : Constant  Value=65535  OutDataTypeStr=Inherit: Inherit via back propagation
  Rate Transition : RateTransition  Deterministic=off  OutPortSampleTime=.0005*200
  Switch : Switch  Criteria=u2 ~= 0  SaturateOnIntegerOverflow=off  InputSameDT=off
  CPU Load : Outport  Unit=%  SampleTime=.0005*200
  CPU Overload : Outport  Port=2
  wires:
  Rate Transition/1 -> Switch/2
  MCU Overload/1 -> Rate Transition/1, CPU Overload/1
  MCU Load/1 -> Downsample Averaged2/1(In1)
  Downsample Averaged2/1(Out1) -> Switch/3
  Switch/1 -> Gain/1
  Overload/1 -> Switch/1
  Gain/1 -> CPU Load/1

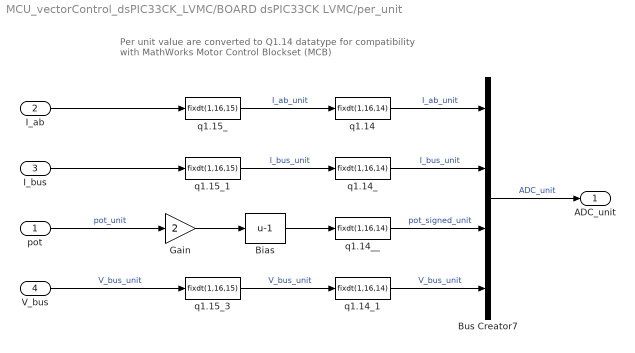
== system MCU_vectorControl_dsPIC33CK_LVMC/BOARD dsPIC33CK LVMC/per_unit ==
  note: Per unit value are converted to Q1.14 datatype
      | for compatibility with MathWorks Motor Control Blockset (MCB)
  pot : Inport
  I_ab : Inport  Port=2
  I_bus : Inport  Port=3
  V_bus : Inport  Port=4
  Bias : Bias  Bias=-1  SaturateOnIntegerOverflow=off
  Bus Creator7 : BusCreator  Inputs=4
  Gain : Gain  Gain=2  OutDataTypeStr=fixdt(1,16,15)  LockScale=on
  q1.14 : DataTypeConversion  OutDataTypeStr=fixdt(1,16,14)  SaturateOnIntegerOverflow=off  RndMeth=Floor  LockScale=on
  q1.14_ : DataTypeConversion  OutDataTypeStr=fixdt(1,16,14)  SaturateOnIntegerOverflow=off  RndMeth=Floor  LockScale=on
  q1.14_1 : DataTypeConversion  OutDataTypeStr=fixdt(1,16,14)  SaturateOnIntegerOverflow=off  RndMeth=Floor  LockScale=on
  q1.14__ : DataTypeConversion  OutDataTypeStr=fixdt(1,16,14)  SaturateOnIntegerOverflow=off  RndMeth=Floor  LockScale=on
  q1.15_ : DataTypeConversion  OutDataTypeStr=fixdt(1,16,15)  ConvertRealWorld=Stored Integer (SI)  SaturateOnIntegerOverflow=off  RndMeth=Floor  LockScale=on
  q1.15_1 : DataTypeConversion  OutDataTypeStr=fixdt(1,16,15)  ConvertRealWorld=Stored Integer (SI)  SaturateOnIntegerOverflow=off  RndMeth=Floor  LockScale=on
  q1.15_3 : DataTypeConversion  OutDataTypeStr=fixdt(1,16,15)  ConvertRealWorld=Stored Integer (SI)  SaturateOnIntegerOverflow=off  RndMeth=Floor  LockScale=on
  ADC_unit : Outport
  wires:
  I_ab/1 -> q1.15_/1
  V_bus/1 -> q1.15_3/1  "V_bus_unit"
  pot/1 -> Gain/1  "pot_unit"
  I_bus/1 -> q1.15_1/1
  q1.15_1/1 -> q1.14_/1  "I_bus_unit"
  q1.15_/1 -> q1.14/1  "I_ab_unit"
  Bus Creator7/1 -> ADC_unit/1  "ADC_unit"
  q1.15_3/1 -> q1.14_1/1  "V_bus_unit"
  q1.14/1 -> Bus Creator7/1  "I_ab_unit"
  q1.14_/1 -> Bus Creator7/2  "I_bus_unit"
  q1.14__/1 -> Bus Creator7/3  "pot_signed_unit"
  q1.14_1/1 -> Bus Creator7/4  "V_bus_unit"
  Gain/1 -> Bias/1
  Bias/1 -> q1.14__/1

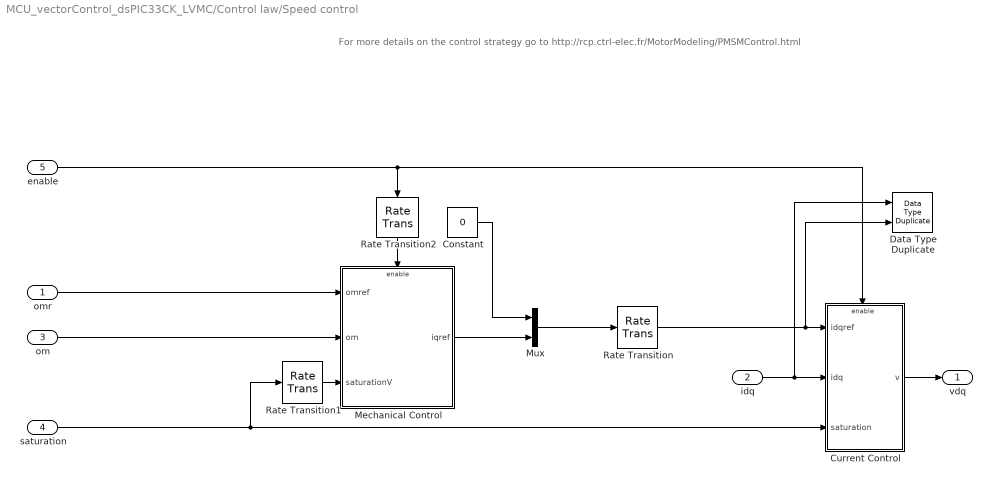
== system MCU_vectorControl_dsPIC33CK_LVMC/Control law/Speed control ==
  note: For more details on the control strategy go to
      |
      | http://rcp.ctrl-elec.fr/MotorModeling/PMSMControl.html
  omr : Inport
  idq : Inport  Port=2
  om : Inport  Port=3
  saturation : Inport  Port=4
  enable : Inport  Port=5
  Constant : Constant  Value=0  OutDataTypeStr=Inherit: Inherit via back propagation
  Current Control : Subsystem
  Data Type Duplicate : DataTypeDuplicate
  Mechanical Control : Subsystem
  Mux : Mux  Inputs=2
  Rate Transition : RateTransition
  Rate Transition1 : RateTransition  OutPortSampleTime=control.tsMeca
  Rate Transition2 : RateTransition
  vdq : Outport
  wires:
  idq/1 -> Data Type Duplicate/1, Current Control/2(idq)
  Mux/1 -> Rate Transition/1
  Current Control/1(v) -> vdq/1
  saturation/1 -> Rate Transition1/1, Current Control/3(saturation)
  om/1 -> Mechanical Control/2(om)
  Constant/1 -> Mux/1
  Mechanical Control/1(iqref) -> Mux/2
  Rate Transition/1 -> Data Type Duplicate/2, Current Control/1(idqref)
  omr/1 -> Mechanical Control/1(omref)
  Rate Transition1/1 -> Mechanical Control/3(saturationV)
  enable/1 -> Current Control/Enable, Rate Transition2/1
  Rate Transition2/1 -> Mechanical Control/Enable

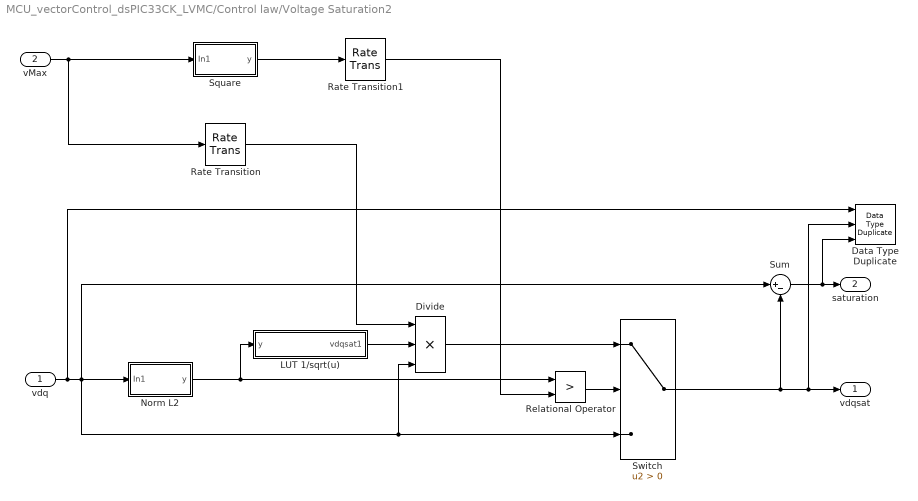
== system MCU_vectorControl_dsPIC33CK_LVMC/Control law/Voltage Saturation2 ==
  vdq : Inport
  vMax : Inport  Port=2
  Data Type Duplicate : DataTypeDuplicate  NumInputPorts=3
  Divide : Product  Inputs=***  OutDataTypeStr=Inherit: Inherit via back propagation  SaturateOnIntegerOverflow=on
  "LUT 1/sqrt(u) " : Subsystem
  Norm L2 : Subsystem
  Rate Transition : RateTransition
  Rate Transition1 : RateTransition
  Relational Operator : RelationalOperator  Operator=>  OutDataTypeStr=boolean  RndMeth=Simplest  InputSameDT=off
  Square : Subsystem
  Sum : Sum  Inputs=|+-  OutDataTypeStr=Inherit: Inherit via back propagation  SaturateOnIntegerOverflow=on
  Switch : Switch  Criteria=u2 > Threshold  OutDataTypeStr=Inherit: Inherit via back propagation  SaturateOnIntegerOverflow=off  InputSameDT=off
  vdqsat : Outport  VectorParamsAs1DForOutWhenUnconnected=off
  saturation : Outport  Port=2  VectorParamsAs1DForOutWhenUnconnected=off
  wires:
  "LUT 1/sqrt(u) "/1(vdqsat1) -> Divide/2
  Divide/1 -> Switch/1
  Norm L2/1(y) -> Relational Operator/1, "LUT 1/sqrt(u) "/1(y)
  Switch/1 -> vdqsat/1, Data Type Duplicate/2, Sum/2
  vdq/1 -> Sum/1, Switch/3, Divide/3, Norm L2/1(In1), Data Type Duplicate/1
  Sum/1 -> saturation/1, Data Type Duplicate/3
  Relational Operator/1 -> Switch/2
  vMax/1 -> Square/1(In1), Rate Transition/1
  Square/1(y) -> Rate Transition1/1
  Rate Transition/1 -> Divide/1
  Rate Transition1/1 -> Relational Operator/2

== system MCU_vectorControl_dsPIC33CK_LVMC/Control law/off1 ==
  Mux : Mux  Inputs=2
  vd : Constant  Value=0  OutDataTypeStr=Inherit: Inherit via back propagation
  vq : Constant  Value=0  OutDataTypeStr=Inherit: Inherit via back propagation
  vdq : Outport  VectorParamsAs1DForOutWhenUnconnected=off
  wires:
  vd/1 -> Mux/1
  Mux/1 -> vdq/1
  vq/1 -> Mux/2

== system MCU_vectorControl_dsPIC33CK_LVMC/Control law/open loop ==
  vdqr : Inport
  Enable : EnablePort
  vdq : Outport  VectorParamsAs1DForOutWhenUnconnected=off
  wires:
  vdqr/1 -> vdq/1

== system MCU_vectorControl_dsPIC33CK_LVMC/Init Enc/Wait 1s ==
  Enable : EnablePort  StatesWhenEnabling=reset
  AND : Logic  IconShape=distinctive  AllPortsSameDT=off  OutDataTypeStr=boolean
  Compare To Constant : simulink/Logic and Bit Operations/Compare To Constant  relop=>  const=1  OutDataTypeStr=boolean
  Compare To Constant1 : simulink/Logic and Bit Operations/Compare To Constant  relop=>  const=1.1  OutDataTypeStr=boolean
  Constant1 : Constant  OutDataTypeStr=int16
  Discrete-Time Integrator : DiscreteIntegrator  SampleTime=-1  SaturateOnIntegerOverflow=on  LimitOutput=on  UpperSaturationLimit=2  LowerSaturationLimit=0  ICPrevOutput=DiscIntNeverNeededParam  ICPrevScaledInput=DiscIntNeverNeededParam
  NOT : Logic  Operator=NOT  IconShape=distinctive  AllPortsSameDT=off  OutDataTypeStr=boolean
  init enc : Outport
  init done : Outport  Port=2
  wires:
  NOT/1 -> AND/2
  AND/1 -> init enc/1
  Compare To Constant1/1 -> NOT/1, init done/1
  Discrete-Time Integrator/1 -> Compare To Constant/1, Compare To Constant1/1
  Constant1/1 -> Discrete-Time Integrator/1
  Compare To Constant/1 -> AND/1

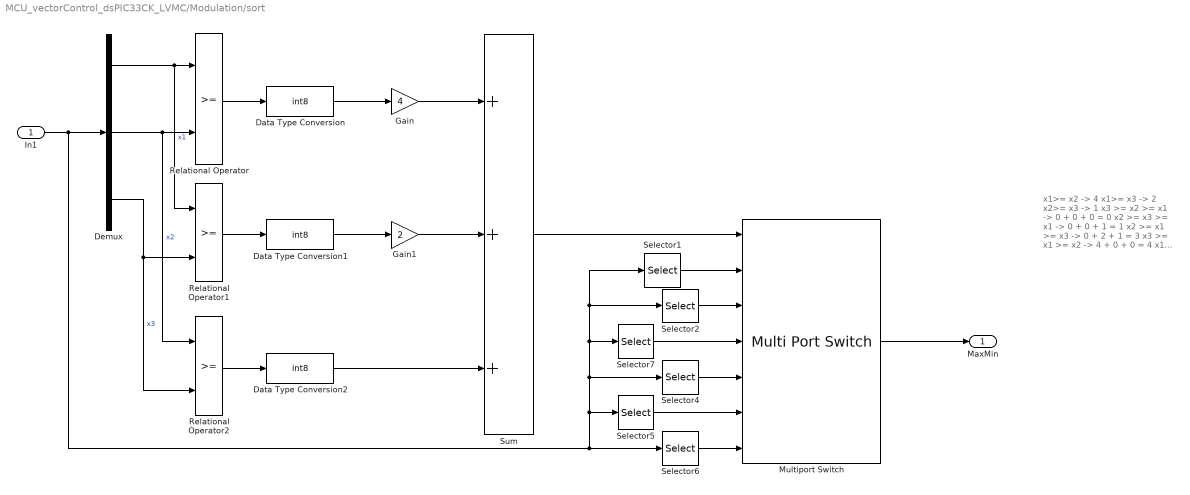
== system MCU_vectorControl_dsPIC33CK_LVMC/Modulation/sort ==
  note: x1>= x2 -> 4
      | x1>= x3 -> 2
      | x2>= x3 -> 1
      |
      | x3 >= x2 >= x1 -> 0 + 0 + 0 = 0
      | x2 >= x3 >= x1 -> 0 + 0 + 1 = 1
      | x2 >= x1 >= x3 -> 0 + 2 + 1 = 3
      | x3 >= x1 >= x2 -> 4 + 0 + 0 = 4
      | x1 >= x3 >= x2 -> 4 + 2 + 0 = 6
      | x1 >= x2 >= x3 -> 4 + 2 + 1 = 7
  In1 : Inport
  Data Type Conversion : DataTypeConversion  OutDataTypeStr=int8  SaturateOnIntegerOverflow=off  RndMeth=Floor
  Data Type Conversion1 : DataTypeConversion  OutDataTypeStr=int8  SaturateOnIntegerOverflow=off  RndMeth=Floor
  Data Type Conversion2 : DataTypeConversion  OutDataTypeStr=int8  SaturateOnIntegerOverflow=off  RndMeth=Floor
  Demux : Demux  Outputs=3
  Gain : Gain  Gain=4  OutDataTypeStr=Inherit: Same as input
  Gain1 : Gain  Gain=2  OutDataTypeStr=Inherit: Same as input
  Multiport Switch : MultiPortSwitch  DataPortOrder=Specify indices  DataPortIndices={0,1,3,4,6,7}  SaturateOnIntegerOverflow=off  InputSameDT=off
  Relational Operator : RelationalOperator  OutDataTypeStr=boolean  RndMeth=Simplest  InputSameDT=off
  Relational Operator1 : RelationalOperator  OutDataTypeStr=boolean  RndMeth=Simplest  InputSameDT=off
  Relational Operator2 : RelationalOperator  OutDataTypeStr=boolean  RndMeth=Simplest  InputSameDT=off
  Selector1 : Selector  InputPortWidth=3  IndexOptions=Index vector (dialog)  Indices=[3 1]  OutputSizes=1
  Selector2 : Selector  InputPortWidth=3  IndexOptions=Index vector (dialog)  Indices=[2 1]  OutputSizes=1
  Selector4 : Selector  InputPortWidth=3  IndexOptions=Index vector (dialog)  Indices=[3 2]  OutputSizes=1
  Selector5 : Selector  InputPortWidth=3  IndexOptions=Index vector (dialog)  Indices=[1 2]  OutputSizes=1
  Selector6 : Selector  InputPortWidth=3  IndexOptions=Index vector (dialog)  Indices=[1 3]  OutputSizes=1
  Selector7 : Selector  InputPortWidth=3  IndexOptions=Index vector (dialog)  Indices=[2 3]  OutputSizes=1
  Sum : Sum  Inputs=+++
  MaxMin : Outport
  wires:
  Demux/3 -> Relational Operator2/2, Relational Operator1/2  "x3"
  Demux/2 -> Relational Operator2/1, Relational Operator/2  "x2"
  Demux/1 -> Relational Operator1/1, Relational Operator/1  "x1"
  In1/1 -> Selector4/1, Selector7/1, Selector2/1, Selector1/1, Selector5/1, Selector6/1, Demux/1
  Relational Operator2/1 -> Data Type Conversion2/1
  Relational Operator1/1 -> Data Type Conversion1/1
  Relational Operator/1 -> Data Type Conversion/1
  Data Type Conversion/1 -> Gain/1
  Data Type Conversion1/1 -> Gain1/1
  Gain1/1 -> Sum/2
  Gain/1 -> Sum/1
  Data Type Conversion2/1 -> Sum/3
  Sum/1 -> Multiport Switch/1
  Selector1/1 -> Multiport Switch/2
  Selector6/1 -> Multiport Switch/7
  Selector5/1 -> Multiport Switch/6
  Selector4/1 -> Multiport Switch/5
  Selector7/1 -> Multiport Switch/4
  Selector2/1 -> Multiport Switch/3
  Multiport Switch/1 -> MaxMin/1

== system MCU_vectorControl_dsPIC33CK_LVMC/Park/Clarke ==
  note: Clark transform
      | $x_{\alpha\beta} = \frac{2}{3}\underbrace{\left[\begin{array}{ccc}1&-\frac{1}{2}&-\frac{1}{2}\\0&\frac{\sqrt{3}}{2}&-\frac{\sqrt{3}}{2}\end{array}\right]}_{C_{23}}x_{abc}$
      | if only 2 currents are measured since $x_a+x_b+x_c = 0$
      | $x_{abc} = \left[\begin{array}{cc}1 & 0\\0 & 1\\-1&-1\end{array}\right]x_{ab}$
      | leading to
      | $x_{\alpha\beta} = \underbrace{\left[\begin{array}{cc}1&0\\\frac{1}{\sqrt{3}}&\frac{2}{\sqrt{3}}\end{array}\right]}_{C_{22}}x_{ab}$
  xab(c) : Inport
  C1 : Gain  Gain=[1/sqrt(3) 2/sqrt(3)]  Multiplication=Matrix(K*u)  OutDataTypeStr=Inherit: Same as input
  Mux : Mux  Inputs=2
  Selector : Selector  InputPortWidth=2  IndexOptions=Index vector (dialog)  Indices=[1]  OutputSizes=1
  xalphabeta : Outport  VectorParamsAs1DForOutWhenUnconnected=off
  wires:
  C1/1 -> Mux/2
  Selector/1 -> Mux/1
  Mux/1 -> xalphabeta/1
  xab(c)/1 -> C1/1, Selector/1

== system MCU_vectorControl_dsPIC33CK_LVMC/Park/Park ==
  note: Park
      | $x_{dq} = P(\theta)^{-1}x_{\alpha\beta}\\ P(p\theta)^{-1} = \left[\begin{array}{cc}\cos(p\theta) & \sin(p\theta)\\ -\sin(p\theta) & \cos(p\theta) \end{array}\right]$
  xalphabeta : Inport  PortDimensions=2
  P(pth) : Inport  Port=2
  Data Type Duplicate2 : DataTypeDuplicate
  Park : Product  Multiplication=Matrix(*)  OutDataTypeStr=Inherit: Inherit via back propagation  RndMeth=Round
  xdq : Outport  VectorParamsAs1DForOutWhenUnconnected=off
  wires:
  P(pth)/1 -> Park/1
  xalphabeta/1 -> Park/2, Data Type Duplicate2/2
  Park/1 -> xdq/1, Data Type Duplicate2/1

== system MCU_vectorControl_dsPIC33CK_LVMC/Park inverse/Clarke Inverse ==
  note: Clarke inverse
  xalphabeta : Inport
  C23' : Gain  Gain=|  Multiplication=Matrix(K*u)  OutDataTypeStr=Inherit: Inherit via back propagation  RndMeth=Round
      | [1   -1/2        -1/2;
      |         0   sqrt(3)/2   -sqrt(3)/2]'
  xabc : Outport  VectorParamsAs1DForOutWhenUnconnected=off
  wires:
  xalphabeta/1 -> C23'/1
  C23'/1 -> xabc/1
